simulink model "Lab1_Simulink_model"  (R2019b)
settings: Solver=ode45  StartTime=0.0  StopTime=N*Ts  RelTol=1e-3
values from neighbouring files (symbols this model uses):
  ampl = 0.45    [Lab1.m]    (also in Lab2.m; Question_4_Differential.m)
  offset = 0.5    [Lab1.m]    (also in Lab2.m; Question_4_Differential.m)
libraries: simulink_extras x1, dspsigops x1
settings Model: Creator=David  LastModifiedBy=david.rivera
settings DataIOCC: ReturnWorkspaceOutputs=off
settings DebuggingCC: ArithmeticOperatorsInVariantConditions=warning
settings SFSimCC: SimUseLocalCustomCode=off  CustomCodeUndefinedFunction=UseInterfaceOnly
settings RTWCC: RTWUseLocalCustomCode=off

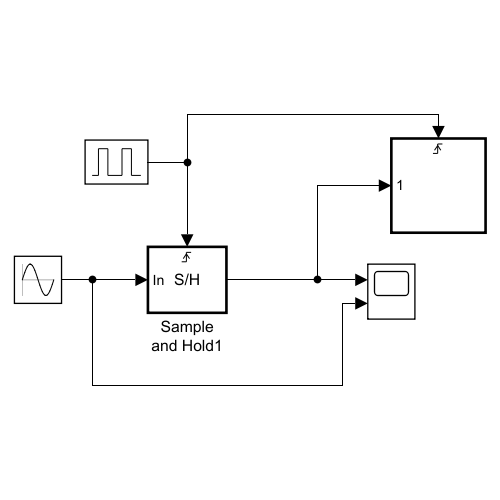
[thumbnail: Simulink's stored preview of the top-level diagram]
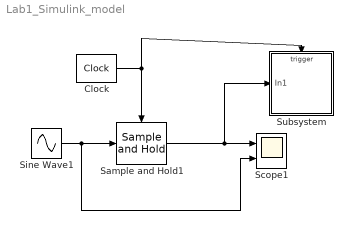
== system Lab1_Simulink_model ==
  Clock : simulink_extras/Flip Flops/Clock  period=Ts
  Sample and Hold1 : dspsigops/Sample and Hold  trig=Rising edge  initCond=0  latchinput=off
  Scope1 : Scope  NumInputPorts=2
  Sine Wave1 : Sin  Amplitude=ampl  Bias=offset  Frequency=2*pi*fi  SampleTime=0
  Subsystem : Subsystem
  wires:
  Sine Wave1/1 -> Scope1/2, Sample and Hold1/1
  Sample and Hold1/1 -> Subsystem/1(In1), Scope1/1
  Clock/1 -> Subsystem/Trigger, Sample and Hold1/Trigger

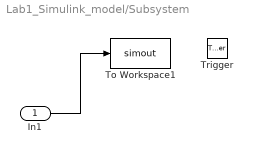
== system Lab1_Simulink_model/Subsystem ==
  In1 : Inport
  Trigger : TriggerPort  VariantControl=Variant  PortDimensions=1
  To Workspace1 : ToWorkspace  VariableName=simout  SampleTime=-1
      settings: Save2DSignal=2-D array (concatenate along first dimension)
  wires:
  In1/1 -> To Workspace1/1
